simulink model "Model"  (R2020b)
settings: Solver=FixedStepAuto  StartTime=0.0  StopTime=10  RelTol=1e-3
values from neighbouring files (symbols this model uses):
  A = [0 1 0 0; -K/m -D/m 0 0;0 0 0 1;0 0 0 -R/L]    [Proiect.m]
  Ad2 = eye(4) +Te*A    [Proiect.m]
  B = [0 0;0 1/m;0 0;1/L 0]    [Proiect.m]
  Bd2 = Te*B    [Proiect.m]
  C = [1 0 0 0;0 0 1 0;0 1 0 0]    [Proiect.m]
  Fx = inv(C*inv(-A + B*K_control)*B)    [Proiect.m]
  K_control = (place(A,B,[-1 -10 -0.5 -20]))    [Proiect.m]
  K_control_dis2 = (place(Ad2,Bd2,pDis))    [Proiect.m]
  K_es_dis2 = ((place(Ad2',C',pDis_des2)))    [Proiect.m]
  sysD = c2d(sysC,Te,'zoh')    [Proiect.m]
  Te = 1/2000    (= 0.0005)    [Proiect.m]
undefined symbols (not defined in the file or in its folder): DiscIntNeverNeededParam, Fx_dis, K_control_dis
settings Model: Creator=Castoleru  LastModifiedBy=Castoleru

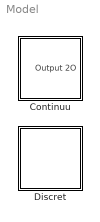
== system Model ==
  Continuu : Subsystem
  Discret : Subsystem

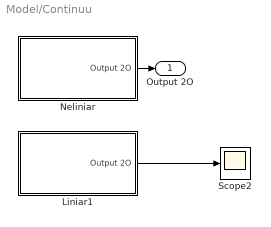
== system Model/Continuu ==
  Liniar1 : Subsystem
  Neliniar : Subsystem
  Scope2 : Scope
  Output 2O : Outport
  wires:
  Liniar1/1(Output 2O) -> Scope2/1
  Neliniar/1(Output 2O) -> Output 2O/1

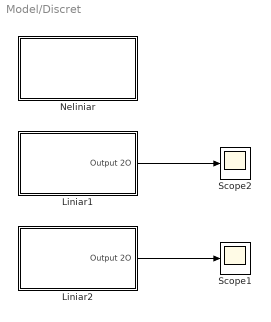
== system Model/Discret ==
  Liniar1 : Subsystem
  Liniar2 : Subsystem
  Neliniar : Subsystem
  Scope1 : Scope
  Scope2 : Scope
  wires:
  Liniar1/1(Output 2O) -> Scope2/1
  Liniar2/1(Output 2O) -> Scope1/1

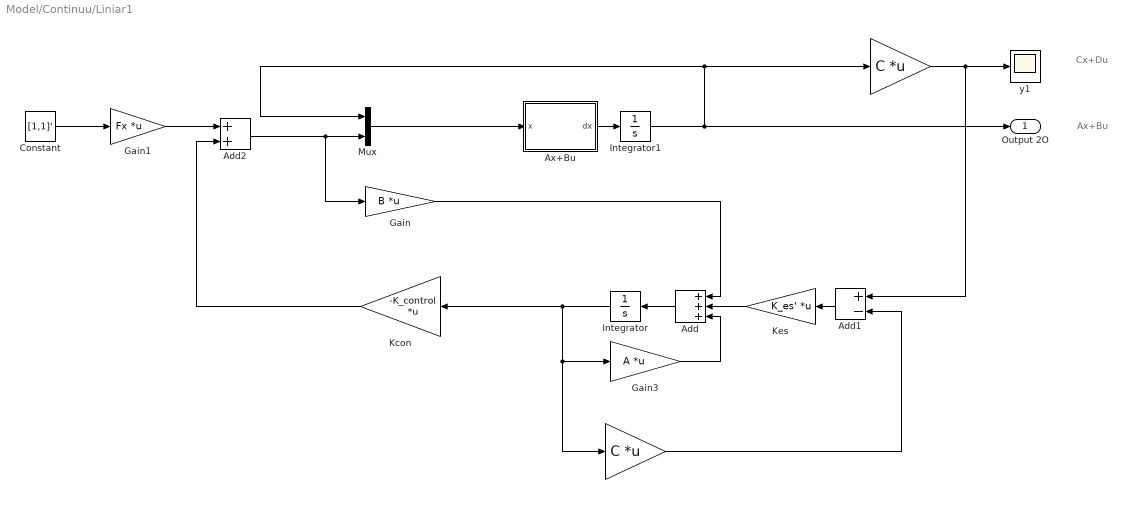
== system Model/Continuu/Liniar1 ==
  note: Cx+Du
  note: Ax+Bu
  " " : Gain  Gain=C  Multiplication=Matrix(K*u) (u vector)
  "  " : Gain  Gain=C  Multiplication=Matrix(K*u) (u vector)
  Add : Sum  Inputs=+++
  Add1 : Sum  Inputs=+-
  Add2 : Sum
  Ax+Bu : MATLAB Function  TreatAsAtomicUnit=on
  Constant : Constant  Value=[1,1]'
  Gain : Gain  Gain=B  Multiplication=Matrix(K*u) (u vector)
  Gain1 : Gain  Gain=Fx  Multiplication=Matrix(K*u) (u vector)
  Gain3 : Gain  Gain=A  Multiplication=Matrix(K*u) (u vector)
  Integrator : Integrator  InitialCondition=[0,0,0,0]'
  Integrator1 : Integrator  InitialCondition=[0.1,0.5,0.25,-0.5]'
  Kcon : Gain  Gain=-K_control  Multiplication=Matrix(K*u) (u vector)
  Kes : Gain  Gain=K_es'  Multiplication=Matrix(K*u) (u vector)
  Mux : Mux  Inputs=2
  y1 : Scope
  Output 2O : Outport
  wires:
  Integrator1/1 -> "  "/1, Mux/1, Output 2O/1
  Ax+Bu/1(dx) -> Integrator1/1
  "  "/1 -> Add1/1, y1/1
  Kes/1 -> Add/2
  Gain/1 -> Add/1
  Add/1 -> Integrator/1
  Integrator/1 -> Kcon/1, Gain3/1, " "/1
  Gain3/1 -> Add/3
  Add1/1 -> Kes/1
  " "/1 -> Add1/2
  Mux/1 -> Ax+Bu/1(x)
  Kcon/1 -> Add2/2
  Add2/1 -> Gain/1, Mux/2
  Gain1/1 -> Add2/1
  Constant/1 -> Gain1/1

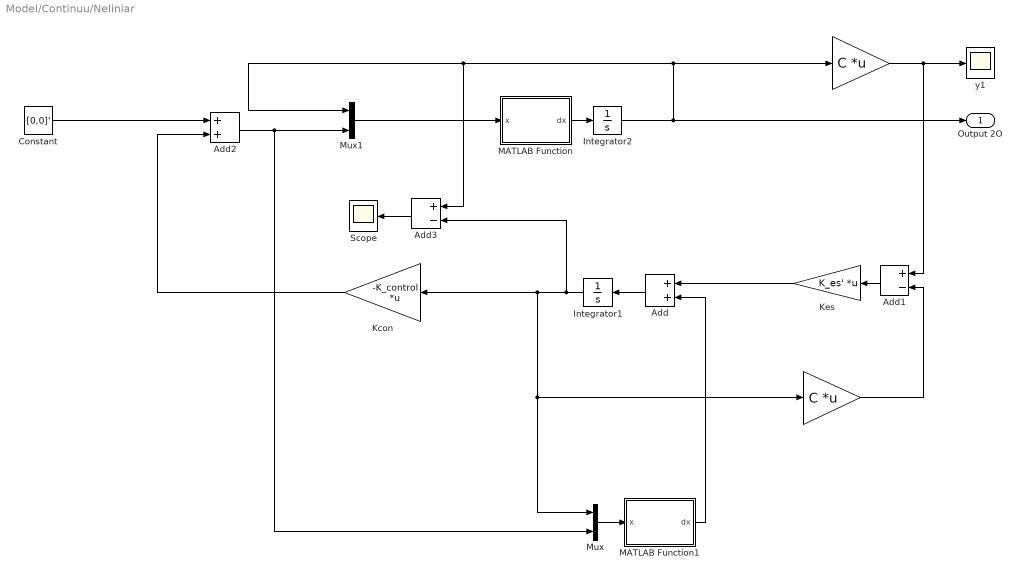
== system Model/Continuu/Neliniar ==
  " " : Gain  Gain=C  Multiplication=Matrix(K*u) (u vector)
  "  " : Gain  Gain=C  Multiplication=Matrix(K*u) (u vector)
  Add : Sum
  Add1 : Sum  Inputs=+-
  Add2 : Sum
  Add3 : Sum  Inputs=+-
  Constant : Constant  Value=[0,0]'
  Integrator1 : Integrator  InitialCondition=[0,0,0,0]'
  Integrator2 : Integrator  InitialCondition=[0.1,0.5,0.25,-0.5]'*1e-10
  Kcon : Gain  Gain=-K_control  Multiplication=Matrix(K*u) (u vector)
  Kes : Gain  Gain=K_es'  Multiplication=Matrix(K*u) (u vector)
  MATLAB Function : MATLAB Function  TreatAsAtomicUnit=on
  MATLAB Function1 : MATLAB Function  TreatAsAtomicUnit=on
  Mux : Mux  Inputs=2
  Mux1 : Mux  Inputs=2
  Scope : Scope
  y1 : Scope
  Output 2O : Outport
  wires:
  Constant/1 -> Add2/1
  Add2/1 -> Mux/2, Mux1/2
  "  "/1 -> Add1/1, y1/1
  " "/1 -> Add1/2
  Mux1/1 -> MATLAB Function/1(x)
  Kcon/1 -> Add2/2
  Add/1 -> Integrator1/1
  MATLAB Function/1(dx) -> Integrator2/1
  Integrator2/1 -> "  "/1, Add3/1, Mux1/1, Output 2O/1
  Integrator1/1 -> Add3/2, Kcon/1, Mux/1, " "/1
  Add1/1 -> Kes/1
  Add3/1 -> Scope/1
  Mux/1 -> MATLAB Function1/1(x)
  Kes/1 -> Add/1
  MATLAB Function1/1(dx) -> Add/2

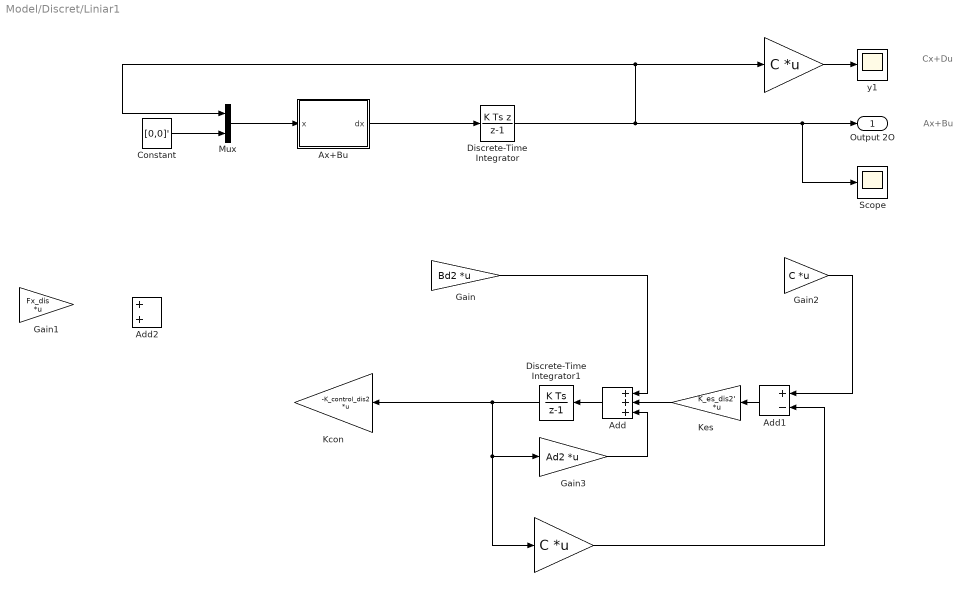
== system Model/Discret/Liniar1 ==
  note: Cx+Du
  note: Ax+Bu
  " " : Gain  Gain=C  Multiplication=Matrix(K*u) (u vector)
  "  " : Gain  Gain=C  Multiplication=Matrix(K*u) (u vector)
  Add : Sum  Inputs=+++
  Add1 : Sum  Inputs=+-
  Add2 : Sum
  Ax+Bu : MATLAB Function  TreatAsAtomicUnit=on
  Constant : Constant  Value=[0,0]'  SampleTime=Te
  Discrete-Time Integrator : DiscreteIntegrator  IntegratorMethod=Integration: Backward Euler  InitialCondition=[1 0.5 -0.2 -1]'  SampleTime=Te  ICPrevOutput=DiscIntNeverNeededParam  ICPrevScaledInput=DiscIntNeverNeededParam
  Discrete-Time Integrator1 : DiscreteIntegrator  InitialCondition=[0 0 0 0]'  SampleTime=Te  ICPrevOutput=DiscIntNeverNeededParam  ICPrevScaledInput=DiscIntNeverNeededParam
  Gain : Gain  Gain=Bd2  Multiplication=Matrix(K*u) (u vector)
  Gain1 : Gain  Gain=Fx_dis  Multiplication=Matrix(K*u) (u vector)
  Gain2 : Gain  Gain=C  Multiplication=Matrix(K*u) (u vector)
  Gain3 : Gain  Gain=Ad2  Multiplication=Matrix(K*u) (u vector)
  Kcon : Gain  Gain=-K_control_dis2  Multiplication=Matrix(K*u) (u vector)
  Kes : Gain  Gain=K_es_dis2'  Multiplication=Matrix(K*u) (u vector)
  Mux : Mux  Inputs=2
  Scope : Scope
  y1 : Scope
  Output 2O : Outport
  wires:
  "  "/1 -> y1/1
  Gain2/1 -> Add1/1
  Discrete-Time Integrator/1 -> Scope/1, Output 2O/1, "  "/1, Mux/1
  Add1/1 -> Kes/1
  Discrete-Time Integrator1/1 -> Kcon/1, Gain3/1, " "/1
  " "/1 -> Add1/2
  Add/1 -> Discrete-Time Integrator1/1
  Gain3/1 -> Add/3
  Gain/1 -> Add/1
  Kes/1 -> Add/2
  Constant/1 -> Mux/2
  Mux/1 -> Ax+Bu/1(x)
  Ax+Bu/1(dx) -> Discrete-Time Integrator/1

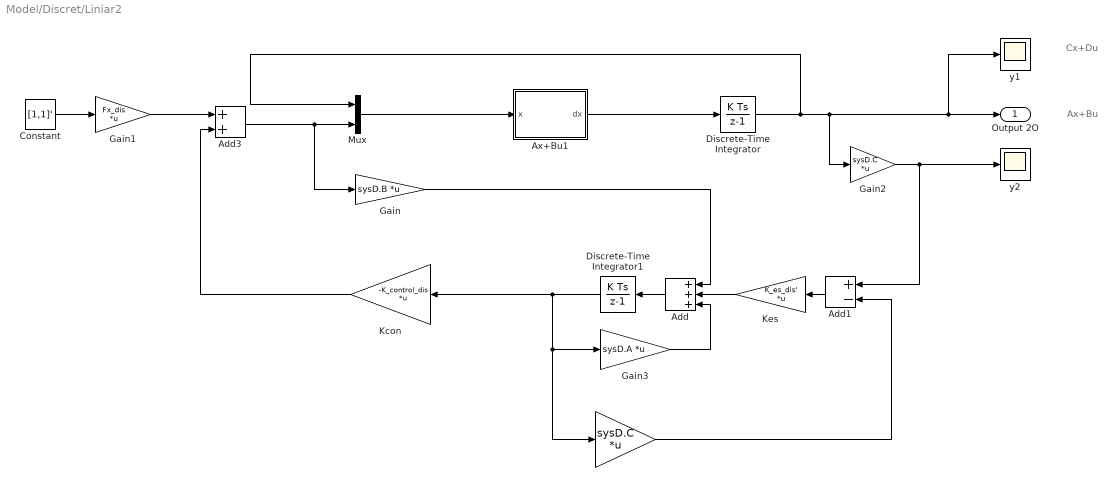
== system Model/Discret/Liniar2 ==
  note: Cx+Du
  note: Ax+Bu
  " " : Gain  Gain=sysD.C  Multiplication=Matrix(K*u) (u vector)
  Add : Sum  Inputs=+++
  Add1 : Sum  Inputs=+-
  Add3 : Sum
  Ax+Bu1 : MATLAB Function  TreatAsAtomicUnit=on
  Constant : Constant  Value=[1,1]'  SampleTime=Te
  Discrete-Time Integrator : DiscreteIntegrator  InitialCondition=[0.3 0.1 -0.1 -0.2]'  SampleTime=Te  ICPrevOutput=DiscIntNeverNeededParam  ICPrevScaledInput=DiscIntNeverNeededParam
  Discrete-Time Integrator1 : DiscreteIntegrator  InitialCondition=[0 0 0 0]'  SampleTime=Te  ICPrevOutput=DiscIntNeverNeededParam  ICPrevScaledInput=DiscIntNeverNeededParam
  Gain : Gain  Gain=sysD.B  Multiplication=Matrix(K*u) (u vector)
  Gain1 : Gain  Gain=Fx_dis  Multiplication=Matrix(K*u) (u vector)
  Gain2 : Gain  Gain=sysD.C  Multiplication=Matrix(K*u) (u vector)
  Gain3 : Gain  Gain=sysD.A  Multiplication=Matrix(K*u) (u vector)
  Kcon : Gain  Gain=-K_control_dis  Multiplication=Matrix(K*u) (u vector)
  Kes : Gain  Gain=K_es_dis'  Multiplication=Matrix(K*u) (u vector)
  Mux : Mux  Inputs=2
  y1 : Scope
  y2 : Scope
  Output 2O : Outport
  wires:
  Kes/1 -> Add/2
  Gain/1 -> Add/1
  Add/1 -> Discrete-Time Integrator1/1
  Discrete-Time Integrator1/1 -> Kcon/1, Gain3/1, " "/1
  Gain3/1 -> Add/3
  Add1/1 -> Kes/1
  " "/1 -> Add1/2
  Mux/1 -> Ax+Bu1/1(x)
  Ax+Bu1/1(dx) -> Discrete-Time Integrator/1
  Discrete-Time Integrator/1 -> Mux/1, Gain2/1, y1/1, Output 2O/1
  Add3/1 -> Gain/1, Mux/2
  Constant/1 -> Gain1/1
  Kcon/1 -> Add3/2
  Gain1/1 -> Add3/1
  Gain2/1 -> Add1/1, y2/1

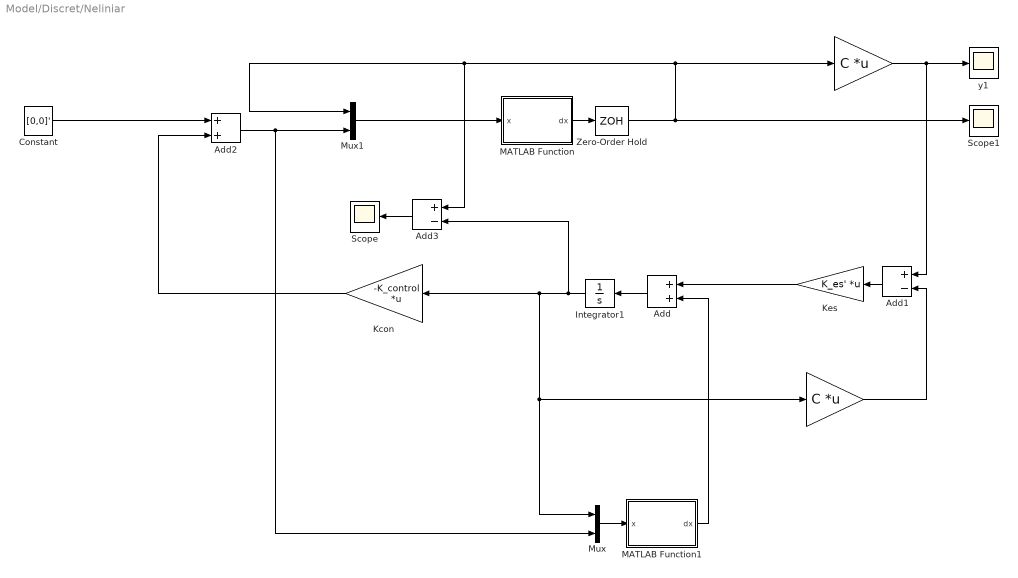
== system Model/Discret/Neliniar ==
  " " : Gain  Gain=C  Multiplication=Matrix(K*u) (u vector)
  "  " : Gain  Gain=C  Multiplication=Matrix(K*u) (u vector)
  Add : Sum
  Add1 : Sum  Inputs=+-
  Add2 : Sum
  Add3 : Sum  Inputs=+-
  Constant : Constant  Value=[0,0]'
  Integrator1 : Integrator  InitialCondition=[0,0,0,0]'
  Kcon : Gain  Gain=-K_control  Multiplication=Matrix(K*u) (u vector)
  Kes : Gain  Gain=K_es'  Multiplication=Matrix(K*u) (u vector)
  MATLAB Function : MATLAB Function  TreatAsAtomicUnit=on
  MATLAB Function1 : MATLAB Function  TreatAsAtomicUnit=on
  Mux : Mux  Inputs=2
  Mux1 : Mux  Inputs=2
  Scope : Scope
  Scope1 : Scope
  Zero-Order Hold : ZeroOrderHold  SampleTime=-1
  y1 : Scope
  wires:
  Constant/1 -> Add2/1
  Add2/1 -> Mux/2, Mux1/2
  "  "/1 -> Add1/1, y1/1
  " "/1 -> Add1/2
  Mux1/1 -> MATLAB Function/1(x)
  Kcon/1 -> Add2/2
  Add/1 -> Integrator1/1
  MATLAB Function/1(dx) -> Zero-Order Hold/1
  Zero-Order Hold/1 -> Scope1/1, "  "/1, Add3/1, Mux1/1
  Integrator1/1 -> Add3/2, Kcon/1, Mux/1, " "/1
  Add1/1 -> Kes/1
  Add3/1 -> Scope/1
  Mux/1 -> MATLAB Function1/1(x)
  Kes/1 -> Add/1
  MATLAB Function1/1(dx) -> Add/2

== matlab function Model/Continuu/Neliniar/MATLAB Function ==
  data: x input; dx output
function dx = fcn(x)
R = 2e6  
L = 1e4 
m = 0.1
K = 10 
D = 10 
epsilon = 10e-6 * 8.854 
A = 2* 10e-2 
alpha = epsilon * A 
beta = 0.005 
% x(5) = E
% x(6) = Fext;
dx = [x(2),...
     (x(6)-D*x(2) - K*x(1) - x(3)^2/(2*alpha))/m,...
      x(4),...
     (x(5)-R*x(4)-x(1)*x(3)/alpha)/L]';

== matlab function Model/Continuu/Liniar1/Ax+Bu ==
  data: x input; dx output
function dx = fcn(x)
R = 2e6  
L = 1e4 
m = 0.1
K = 10 
D = 10 
epsilon = 10e-6 * 8.854 
A = 2* 10e-2 
alpha = epsilon * A 
beta = 0.005 
% x(5) = E
% x(6) = Fext;
dx = [x(2),...
     (x(6)-D*x(2) - K*x(1))/m,...
      x(4),...
     (x(5)-R*x(4))/L]';
end

== matlab function Model/Discret/Liniar1/Ax+Bu ==
  data: x input; dx output
function dx = fcn(x)
% R = 2e6  
% L = 1e4 
% m = 0.1
% K = 10 
% D = 10 
% epsilon = 10e-6 * 8.854 
% A = 2* 10e-2 
% alpha = epsilon * A 
% beta = 0.005 
% x(5) = E
% x(6) = Fext;
dx = [x(1) + 0.0005 *x(2),...
     -0.0500 *x(1)+0.9500*x(2)+ 0.005*x(6),...
     x(3)+0.0005*x(4),...
     0.9*x(4)+5e-08*x(5)]';
end

== matlab function Model/Discret/Neliniar/MATLAB Function ==
  data: x input; dx output
function dx = fcn(x)
R = 2e6  
L = 1e4 
m = 0.1
K = 10 
D = 10 
epsilon = 10e-6 * 8.854 
A = 2* 10e-2 
alpha = epsilon * A 
beta = 0.005 
% x(5) = E
% x(6) = Fext;
dx = [x(2),...
     (x(6)-D*x(2) - K*x(1) - x(3)^2/(2*alpha))/m,...
      x(4),...
     (x(5)-R*x(4)-x(1)*x(3)/alpha)/L]';

== matlab function Model/Discret/Neliniar/MATLAB Function1 ==
  data: x input; dx output
function dx = fcn(x)
R = 2e6  
L = 1e4 
m = 0.1
K = 10 
D = 10 
epsilon = 10e-6 * 8.854 
A = 2* 10e-2 
alpha = epsilon * A 
beta = 0.005 
% x(5) = E
% x(6) = Fext;
dx = [x(2),...
     (x(6)-D*x(2) - K*x(1) - x(3)^2/(2*alpha))/m,...
      x(4),...
     (x(5)-R*x(4)-x(1)*x(3)/alpha)/L]';

== matlab function Model/Discret/Liniar2/Ax+Bu1 ==
  data: x input; dx output
function dx = fcn(x)
R = 2e6  
L = 1e4 
m = 0.1
K = 10 
D = 10 
epsilon = 10e-6 * 8.854 
A = 2* 10e-2 
alpha = epsilon * A 
beta = 0.005 
% x(5) = E
% x(6) = Fext;
dx = [x(1)+4.877037229727535e-04*x(2)+ 1.229421947987911e-06*x(6),...
     -0.048770372297275*x(1)+0.951217333483245*x(2)+ 0.004877037229728*x(6),...
      x(3)+4.758129098202021e-04*x(4)+ 1.209354508989893e-11*x(5),...
     0.904837418035960*x(4)+ 4.758129098202022e-08*x(5) ]';
end

== matlab function Model/Continuu/Neliniar/MATLAB Function1 ==
  data: x input; dx output
function dx = fcn(x)
R = 2e6  
L = 1e4 
m = 0.1
K = 10 
D = 10 
epsilon = 10e-6 * 8.854 
A = 2* 10e-2 
alpha = epsilon * A 
beta = 0.005 
% x(5) = E
% x(6) = Fext;
dx = [x(2),...
     (x(6)-D*x(2) - K*x(1) - x(3)^2/(2*alpha))/m,...
      x(4),...
     (x(5)-R*x(4)-x(1)*x(3)/alpha)/L]';
